simulink model "Pump2Test"  (R2016b)
settings: Solver=FixedStepAuto  StartTime=0.0  StopTime=simstop  MaxStep=0.1  RelTol=1e-3  EnableMultiTasking=on
values from neighbouring files (symbols this model uses):
  CV01 = 100    [PIDValveTest.m]    (also in PIDtestP2m.m; loggingTest.m)
  simstop = 60*1    (= 60)    [PIDValveTest.m]    (also in PIDtestP2m.m; gatherData.m = WPtime(end)+(WPtime(end)-WPtime(end-1)))
libraries: slrtlib x5, xpcnilib x2, powerlib_meascontrol x1
settings Model: ModifiedByFormat=The MathWorks Inc.  Creator=The MathWorks, Inc.  LastModifiedBy=The MathWorks Inc.
settings SolverCC: EnableConcurrentExecution=on
settings DataIOCC: LimitDataPoints=on  SaveFormat=Array
settings OptimizationCC: BlockReduction=off  DefaultParameterBehavior=Inlined  OptimizeBlockIOStorage=off  BufferReuse=off  GlobalBufferReuse=off  ExpressionFolding=off  ExpressionDepthLimit=2147483647  LocalBlockOutputs=off  LifeSpan=inf
settings DebuggingCC: UnderspecifiedInitializationDetection=Classic  MergeDetectMultiDrivingBlocksExec=none  SolverPrmCheckMsg=warning  FcnCallInpInsideContextMsg=warning  AllowSymbolicDim=off  StateNameClashWarn=warning  SFUnexpectedBacktrackingDiag=warning  SFNoUnconditionalDefaultTransitionDiag=warning  SFExecutionAtInitializationDiag=none
settings HardwareCC: ProdBitPerPointer=32  ProdBitPerSizeT=32  ProdBitPerPtrDiffT=32  ProdLargestAtomicFloat=None  ProdWordSize=32  ProdLongLongMode=on  ProdHWDeviceType=Generic->32-bit x86 compatible
settings ModelReferenceCC: ModelReferenceNumInstancesAllowed=Single  ModelReferenceMinAlgLoopOccurrences=on  PropagateSignalLabelsOutOfModel=off
settings RTWCC: SystemTargetFile=slrt.tlc  TemplateMakefile=slrt_default_tmf  Description=Simulink Real-Time  RTWVerbose=off
settings ConfigComp: CovMetricSettings=dw  CovHtmlReporting=on  CovSaveCumulativeToWorkspaceVar=on  CovSaveSingleToWorkspaceVar=on  CovExternalEMLEnable=off  CovSFcnEnable=off

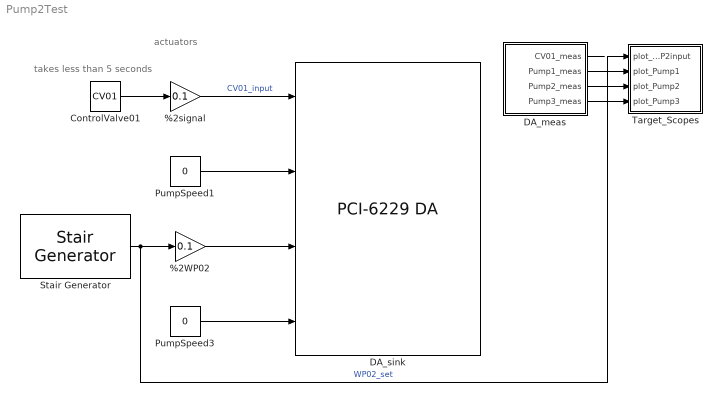
== system Pump2Test ==
  note: takes less than 5 seconds
  note: actuators
  %2WP02 : Gain  Gain=0.1
  %2signal : Gain  Gain=0.1
  ControlValve01 : Constant  Value=CV01
  DA_meas : Subsystem
  DA_sink : xpcnilib/D//A/M Series/PCI-6229 DA  channel=[4 1 2 3]  reset=[1]  initValue=[0]  sampletime=0.01  slot=-1
  PumpSpeed1 : Constant  Value=0
  PumpSpeed3 : Constant  Value=0
  Stair Generator : powerlib_meascontrol/Pulse & Signal Generators/Stair Generator  t=WPtime  e=WP2  Ts=0
  Target_Scopes : Subsystem
  wires:
  PumpSpeed3/1 -> DA_sink/4
  PumpSpeed1/1 -> DA_sink/2
  ControlValve01/1 -> %2signal/1
  DA_meas/2(Pump1_meas) -> Target_Scopes/2(plot_Pump1)
  DA_meas/3(Pump2_meas) -> Target_Scopes/3(plot_Pump2)
  DA_meas/4(Pump3_meas) -> Target_Scopes/4(plot_Pump3)
  DA_meas/1(CV01_meas) -> ?
  %2signal/1 -> DA_sink/1  "CV01_input"
  %2WP02/1 -> DA_sink/3
  Stair Generator/1 -> Target_Scopes/1(plot_WP2input), %2WP02/1  "WP02_set"

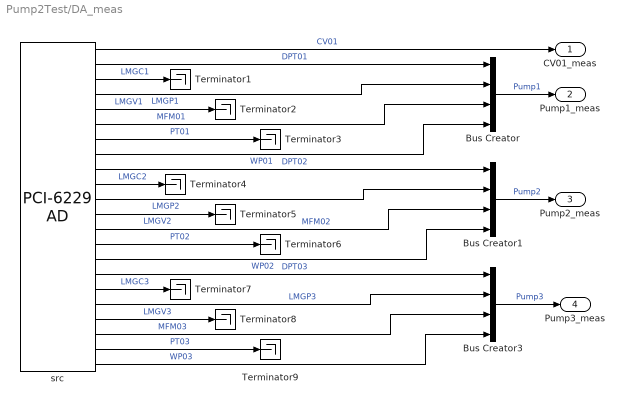
== system Pump2Test/DA_meas ==
  Bus Creator : BusCreator  Inputs=4
  Bus Creator1 : BusCreator  Inputs=4
  Bus Creator3 : BusCreator  Inputs=4
  Terminator{1..9} (9 alike) : Terminator
  src : xpcnilib/A//D/M Series/PCI-6229 AD  channel=[4 17 5 11 8 21 24 1 18 6 12 9 22 25 2 19 7 13 10 23 26 3]  range=[10]  coupling=[0]  scantime=5e-6  sampletime=0.01  slot=-1
  CV01_meas : Outport
  Pump1_meas : Outport  Port=2
  Pump2_meas : Outport  Port=3
  Pump3_meas : Outport  Port=4
  wires:
  Bus Creator/1 -> Pump1_meas/1  "Pump1"
  Bus Creator1/1 -> Pump2_meas/1  "Pump2"
  Bus Creator3/1 -> Pump3_meas/1  "Pump3"
  src/8 -> Bus Creator/4  "WP01"
  src/9 -> Bus Creator1/1  "DPT02"
  src/10 -> Terminator4/1  "LMGC2"
  src/4 -> Bus Creator/2  "LMGP1"
  src/6 -> Bus Creator/3  "MFM01"
  src/7 -> Terminator3/1  "PT01"
  src/2 -> Bus Creator/1  "DPT01"
  src/1 -> CV01_meas/1  "CV01"
  src/3 -> Terminator1/1  "LMGC1"
  src/5 -> Terminator2/1  "LMGV1"
  src/11 -> Bus Creator1/2  "LMGP2"
  src/12 -> Terminator5/1  "LMGV2"
  src/19 -> Terminator8/1  "LMGV3"
  src/17 -> Terminator7/1  "LMGC3"
  src/20 -> Bus Creator3/3  "MFM03"
  src/14 -> Terminator6/1  "PT02"
  src/15 -> Bus Creator1/4  "WP02"
  src/16 -> Bus Creator3/1  "DPT03"
  src/18 -> Bus Creator3/2  "LMGP3"
  src/13 -> Bus Creator1/3  "MFM02"
  src/21 -> Terminator9/1  "PT03"
  src/22 -> Bus Creator3/4  "WP03"

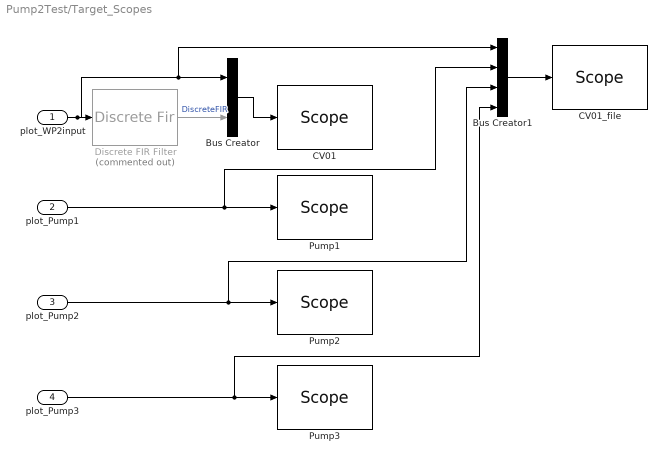
== system Pump2Test/Target_Scopes ==
  plot_WP2input : Inport
  plot_Pump1 : Inport  Port=2
  plot_Pump2 : Inport  Port=3
  plot_Pump3 : Inport  Port=4
  Bus Creator : BusCreator  Inputs=2
  Bus Creator1 : BusCreator  Inputs=4
  CV01 : slrtlib/Displays and Logging/Scope   scopeno=4  scopetype=Target  autostart=on  viewmode=Graphical rolling  formatstr='%15.6f'  grid=on  ylimits=[0,0]  nosamples=simstop*100  noprepostsamples=0  interleave=1  triggermode=FreeRun  triggersignal=1  trigsignalfromport=off  triggerlevel=0.0  triggerslope=Either  triggerscope=1  triggersample=0  filename=data.dat  mode=Lazy  writesize=512  autorestart=off  dynamicfilemode=off  maxwritefilesize=512*1024^2
  CV01_file : slrtlib/Displays and Logging/Scope   scopeno=5  scopetype=File  autostart=on  viewmode=Graphical sliding  formatstr='%15.6f'  grid=on  ylimits=[0,0]  nosamples=100*simstop  noprepostsamples=0  interleave=1  triggermode=FreeRun  triggersignal=1  trigsignalfromport=off  triggerlevel=0.0  triggerslope=Either  triggerscope=1  triggersample=0  filename=E:\3P.dat  mode=Commit  writesize=512  autorestart=off  dynamicfilemode=off  maxwritefilesize=512*1024^2
  Discrete FIR Filter : DiscreteFir  Commented=on  AccumDataTypeStr=Inherit: Same as product output
  Pump1 : slrtlib/Displays and Logging/Scope   scopeno=1  scopetype=Target  autostart=on  viewmode=Graphical sliding  formatstr='%15.6f'  grid=on  ylimits=[0,0]  nosamples=simstop*100  noprepostsamples=0  interleave=1  triggermode=FreeRun  triggersignal=1  trigsignalfromport=off  triggerlevel=0.0  triggerslope=Either  triggerscope=1  triggersample=0  filename=data.dat  mode=Lazy  writesize=512  autorestart=off  dynamicfilemode=off  maxwritefilesize=512*1024^2
  Pump2 : slrtlib/Displays and Logging/Scope   scopeno=2  scopetype=Target  autostart=on  viewmode=Graphical sliding  formatstr='%15.6f'  grid=on  ylimits=[0,0]  nosamples=simstop*100  noprepostsamples=0  interleave=1  triggermode=FreeRun  triggersignal=1  trigsignalfromport=off  triggerlevel=0.0  triggerslope=Either  triggerscope=1  triggersample=0  filename=data.dat  mode=Lazy  writesize=512  autorestart=off  dynamicfilemode=off  maxwritefilesize=512*1024^2
  Pump3 : slrtlib/Displays and Logging/Scope   scopeno=3  scopetype=Target  autostart=on  viewmode=Graphical sliding  formatstr='%15.6f'  grid=on  ylimits=[0,0]  nosamples=simstop*100  noprepostsamples=0  interleave=1  triggermode=FreeRun  triggersignal=1  trigsignalfromport=off  triggerlevel=0.0  triggerslope=Either  triggerscope=1  triggersample=0  filename=data.dat  mode=Lazy  writesize=512  autorestart=off  dynamicfilemode=off  maxwritefilesize=512*1024^2
  wires:
  plot_Pump3/1 -> Bus Creator1/4, Pump3/1
  plot_Pump1/1 -> Bus Creator1/2, Pump1/1
  plot_Pump2/1 -> Bus Creator1/3, Pump2/1
  plot_WP2input/1 -> Bus Creator1/1, Bus Creator/1, Discrete FIR Filter/1
  Bus Creator/1 -> CV01/1
  Discrete FIR Filter/1 -> Bus Creator/2  "DiscreteFIR"
  Bus Creator1/1 -> CV01_file/1
